simulink model "SimpleModel_NL"  (R2013b)
settings: Solver=ode3  StartTime=0.0  StopTime=tend  FixedStep=1e-3  MaxStep=0.1  RelTol=1e-3
undefined symbols (not defined in the file or in its folder): phi
settings Model: Creator=pjseiler  LastModifiedBy=Rodney Dockter
settings DataIOCC: SignalLoggingSaveFormat=ModelDataLogs
settings OptimizationCC: ExpressionDepthLimit=2147483647
settings DebuggingCC: MultiTaskDSMMsg=warning  MultiTaskCondExecSysMsg=none  FcnCallInpInsideContextMsg=EnableAllAsWarning  StateNameClashWarn=warning  StrictBusMsg=None
settings RTWCC: IncludeERTFirstTime=on
settings GRTTargetCC: CodeReplacementLibrary=None  CombineOutputUpdateFcns=off  CPPClassGenCompliant=on  GRTInterface=on

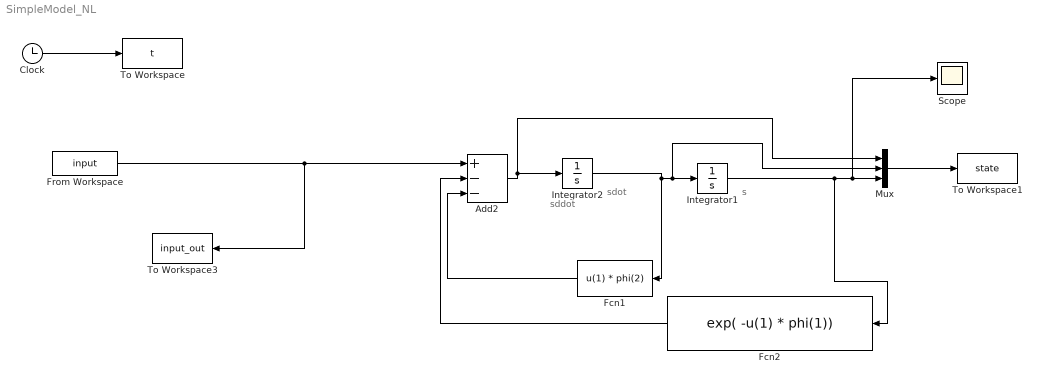
== system SimpleModel_NL ==
  note: sddot
  note: sdot
  note: s
  Add2 : Sum  Inputs=+--
  Clock : Clock
  Fcn1 : Fcn  Expr=u(1) * phi(2)
  Fcn2 : Fcn  Expr=exp( -u(1) * phi(1))
  From Workspace : FromWorkspace  VariableName=input  SampleTime=0
  Integrator1 : Integrator
  Integrator2 : Integrator
  Mux : Mux  Inputs=3
  Scope : Scope
  To Workspace : ToWorkspace  VariableName=t  SampleTime=-1
  To Workspace1 : ToWorkspace  VariableName=state  SampleTime=-1  SaveFormat=Timeseries
  To Workspace3 : ToWorkspace  VariableName=input_out  SampleTime=-1  SaveFormat=Timeseries
  wires:
  Clock/1 -> To Workspace/1
  Integrator2/1 -> Fcn1/1, Integrator1/1, Mux/2
  Integrator1/1 -> Fcn2/1, Mux/3, Scope/1
  Add2/1 -> Integrator2/1, Mux/1
  Fcn1/1 -> Add2/3
  Fcn2/1 -> Add2/2
  Mux/1 -> To Workspace1/1
  From Workspace/1 -> Add2/1, To Workspace3/1
